simulink model "untitled13"  (R2024b)
settings: Solver=VariableStepAuto  StartTime=0.0  StopTime=10.0  RelTol=1e-3
libraries: spsThreePhaseSeriesRLCBranchLib x3, spsThreePhaseVIMeasurementLib x3, spsThreePhaseSourceLib x2, spsThreePhaseParallelRLCLoadLib x1, sps_lib x1
settings Model: Creator=ayush  LastModifiedBy=ayush

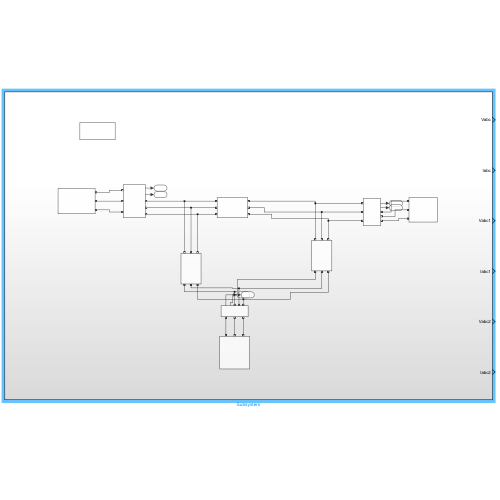
[thumbnail: Simulink's stored preview of the top-level diagram]
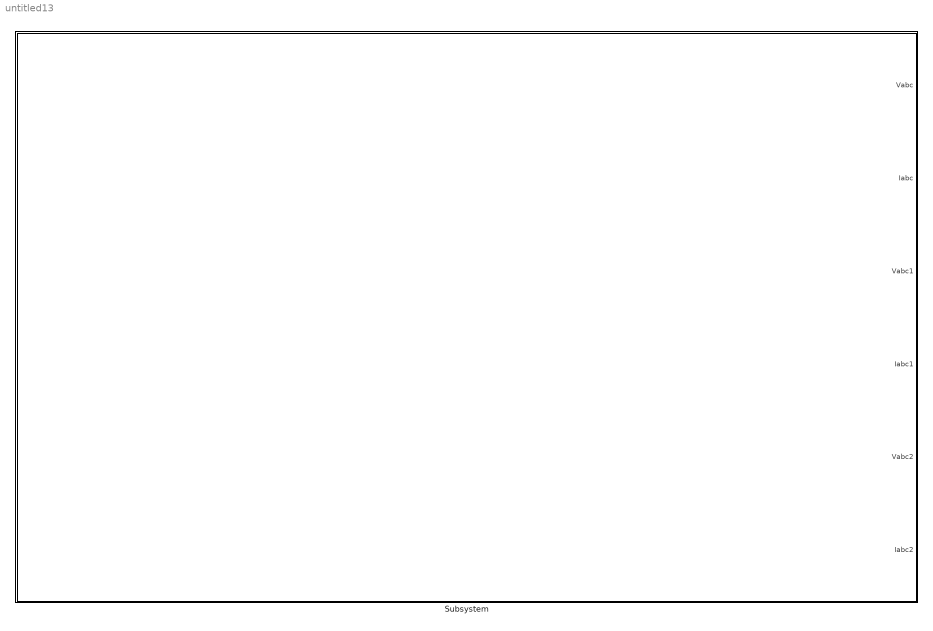
== system untitled13 ==
  Subsystem : Subsystem

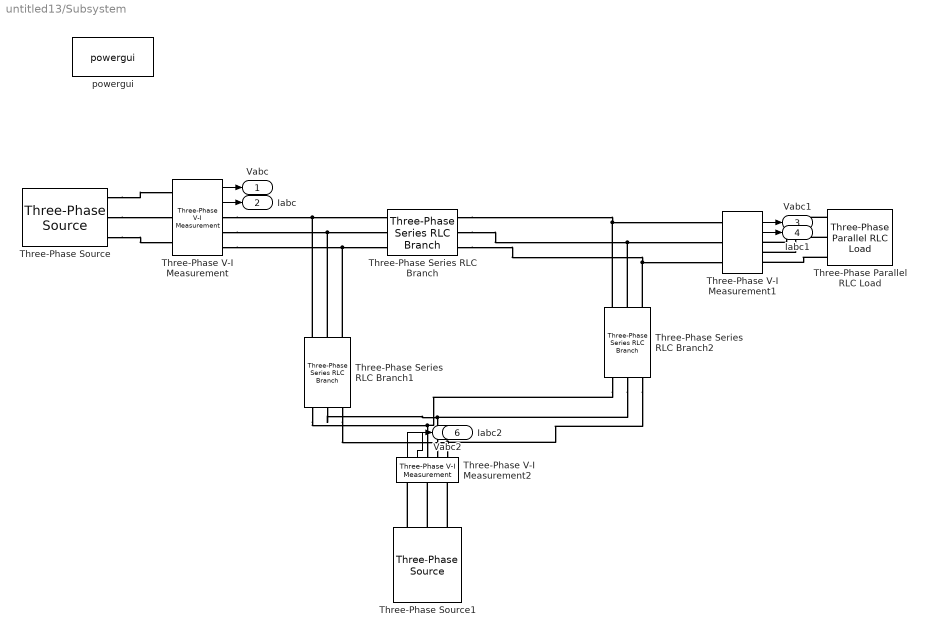
== system untitled13/Subsystem ==
  Three-Phase Parallel RLC Load : spsThreePhaseParallelRLCLoadLib/Three-Phase Parallel RLC Load  LConnTagsString=A|B|C  Configuration=Y (grounded)  NominalVoltage=1000  Vabc=[1e3 1e3 1e3]  Vabcp=[1e3 1e3 1e3]  NominalFrequency=50  UnbalancedPower=off  ActivePower=400e6  InductivePower=250e6  CapacitivePower=0  Pabc=[10e3 9e3 11e3]  QLabc=[100 90 110]  QCabc=[100 90 110]  Pabcp=[10e3 9e3 11e3]  QLabcp=[100 90 110]  QCabcp=[100 90 110]  Measurements=None  LoadType=constant PQ
  Three-Phase Series RLC Branch : spsThreePhaseSeriesRLCBranchLib/Three-Phase Series RLC Branch  LConnTagsString=A|B|C  RConnTagsString=A|B|C  BranchType=RL  Resistance=0.02  Inductance=0.04/(2*3.14*50)  Capacitance=1e-6  Measurements=None
  Three-Phase Series RLC Branch1 : spsThreePhaseSeriesRLCBranchLib/Three-Phase Series RLC Branch  LConnTagsString=A|B|C  RConnTagsString=A|B|C  BranchType=RL  Resistance=1  Inductance=0.03/(2*3.14*50)  Capacitance=1e-6  Measurements=None
  Three-Phase Series RLC Branch2 : spsThreePhaseSeriesRLCBranchLib/Three-Phase Series RLC Branch  LConnTagsString=A|B|C  RConnTagsString=A|B|C  BranchType=RL  Resistance=1  Inductance=0.025/(2*3.14*50)  Capacitance=1e-6  Measurements=None
  Three-Phase V-I Measurement : spsThreePhaseVIMeasurementLib/Three-Phase V-I Measurement  VoltageMeasurement=phase-to-phase  SetLabelV=off  LabelV=Vabc  Vpu=off  VpuLL=off  CurrentMeasurement=yes  SetLabelI=off  LabelI=Iabc  Ipu=off  Pbase=100e6  Vbase=500e3  OutputType=Complex  PhasorSimulation=off  PSBequivalent=0
  Three-Phase V-I Measurement1 : spsThreePhaseVIMeasurementLib/Three-Phase V-I Measurement  VoltageMeasurement=phase-to-phase  SetLabelV=off  LabelV=Vabc  Vpu=off  VpuLL=off  CurrentMeasurement=yes  SetLabelI=off  LabelI=Iabc  Ipu=off  Pbase=100e6  Vbase=500e3  OutputType=Complex  PhasorSimulation=off  PSBequivalent=0
  Three-Phase V-I Measurement2 : spsThreePhaseVIMeasurementLib/Three-Phase V-I Measurement  VoltageMeasurement=phase-to-phase  SetLabelV=off  LabelV=Vabc  Vpu=off  VpuLL=off  CurrentMeasurement=yes  SetLabelI=off  LabelI=Iabc  Ipu=off  Pbase=100e6  Vbase=500e3  OutputType=Complex  PhasorSimulation=off  PSBequivalent=0
  Three-Phase Source : spsThreePhaseSourceLib/Three-Phase Source  InternalConnection=Yg  VoltagePhases=off  Voltage=1.05*10e3  PhaseAngle=0  Voltage_phases=[25e3 25e3 25e3]/sqrt(3)  PhaseAngles_phases=[0 -120 +120]  Frequency=50  NonIdealSource=on  SpecifyImpedance=on  Resistance=0.8929  Inductance=16.58e-3  ShortCircuitLevel=100e6  BaseVoltage=10e3  XRratio=7  BusType=swing  Pref=10e3  Qref=10e6  Prefabc=[10e3, 10e3, 10e3]  Qrefabc=[0, 0, 0]  Qmin=-inf  Qmax=inf
  Three-Phase Source1 : spsThreePhaseSourceLib/Three-Phase Source  InternalConnection=Yg  VoltagePhases=off  Voltage=1.04*10e3  PhaseAngle=0  Voltage_phases=[25e3 25e3 25e3]/sqrt(3)  PhaseAngles_phases=[0 -120 +120]  Frequency=50  NonIdealSource=on  SpecifyImpedance=on  Resistance=0.8929  Inductance=16.58e-3  ShortCircuitLevel=100e6  BaseVoltage=10e3  XRratio=7  BusType=PV  Pref=200e6  Qref=0  Prefabc=[10e3, 10e3, 10e3]  Qrefabc=[0, 0, 0]  Qmin=-inf  Qmax=inf
  powergui : sps_lib/powergui  Priority=1  SimulationMode=Discrete  SampleTime=50e-6  frequency=60  Iterations=50  frequencyindice=50  Pbase=100e6  ErrMax=1e-4  UnitsV=kV  UnitsW=MW  buscounter=0  FunctionMessages=off  echomessages=off  EnableUseOfTLC=off  CurrentSourceSwitches=off  DisableSnubberDevices=off  DisableRonSwitches=off  DisableVfSwitches=off  DisplayEquations=off  AutomaticDiscreteSolvers=off  SolverType=Tustin/Backward Euler (TBE)  Interpol=off  ExternalGateDelay=off  methode=off  Ts=100  x0status=blocks  SPID=on  SwTol=0  HookPort=off  NonlinearTolerance=1e-4  nMaxIteration=100  ContinueOnMaxIteration=off  RestoreLinks=warning  ResistiveCurrentMeasurement=off  Frange=[0:2:500]  Ylog=off  Xlog=on  ShowGrid=off  save=off  variable=ZData  structure=0  ZoomFFT=off  StartTime=0.0  cycles=1  DisplayStyle=1  fundamental=60  FreqAxis=off  MaxFrequency=1000  frequencyindicesteady=1  RmsSteady=1  display=off
  Vabc : Outport
  Iabc : Outport  Port=2
  Vabc1 : Outport  Port=3
  Iabc1 : Outport  Port=4
  Vabc2 : Outport  Port=5
  Iabc2 : Outport  Port=6
  wires:
  Three-Phase V-I Measurement/2 -> Iabc/1
  Three-Phase V-I Measurement1/2 -> Iabc1/1
  Three-Phase V-I Measurement2/1 -> Vabc2/1
  Three-Phase V-I Measurement2/2 -> Iabc2/1
  Three-Phase V-I Measurement1/1 -> Vabc1/1
  Three-Phase V-I Measurement/1 -> Vabc/1
  connections:
  Three-Phase Source/RConn2 -- Three-Phase V-I Measurement/LConn2
  Three-Phase Parallel RLC Load/LConn2 -- Three-Phase V-I Measurement1/RConn2
  Three-Phase V-I Measurement/RConn2 -- Three-Phase Series RLC Branch1/LConn2 -- Three-Phase Series RLC Branch/LConn2
  Three-Phase Series RLC Branch/RConn1 -- Three-Phase Series RLC Branch2/LConn1 -- Three-Phase V-I Measurement1/LConn1
  Three-Phase Series RLC Branch1/RConn2 -- Three-Phase Series RLC Branch2/RConn2 -- Three-Phase V-I Measurement2/RConn2
  Three-Phase Source/RConn1 -- Three-Phase V-I Measurement/LConn1
  Three-Phase Source/RConn3 -- Three-Phase V-I Measurement/LConn3
  Three-Phase Series RLC Branch/RConn2 -- Three-Phase Series RLC Branch2/LConn2 -- Three-Phase V-I Measurement1/LConn2
  Three-Phase Series RLC Branch/RConn3 -- Three-Phase Series RLC Branch2/LConn3 -- Three-Phase V-I Measurement1/LConn3
  Three-Phase V-I Measurement/RConn1 -- Three-Phase Series RLC Branch1/LConn1 -- Three-Phase Series RLC Branch/LConn1
  Three-Phase V-I Measurement/RConn3 -- Three-Phase Series RLC Branch1/LConn3 -- Three-Phase Series RLC Branch/LConn3
  Three-Phase Source1/RConn3 -- Three-Phase V-I Measurement2/LConn3
  Three-Phase Source1/RConn1 -- Three-Phase V-I Measurement2/LConn1
  Three-Phase Series RLC Branch1/RConn1 -- Three-Phase Series RLC Branch2/RConn1 -- Three-Phase V-I Measurement2/RConn1
  Three-Phase Source1/RConn2 -- Three-Phase V-I Measurement2/LConn2
  Three-Phase Parallel RLC Load/LConn3 -- Three-Phase V-I Measurement1/RConn3
  Three-Phase Series RLC Branch1/RConn3 -- Three-Phase Series RLC Branch2/RConn3 -- Three-Phase V-I Measurement2/RConn3
  Three-Phase Parallel RLC Load/LConn1 -- Three-Phase V-I Measurement1/RConn1
